simulink subsystem "ESD"  (R2021a)
settings: Solver=VariableStepAuto  StartTime=0.0  StopTime=10.0  RelTol=1e-3
values from neighbouring files (symbols this model uses):
  params = bestParams    [trainNet.m]
settings Model: Creator=trevor  LastModifiedBy=trevvvy
settings SolverCC: AlgebraicLoopSolver=TrustRegion
settings DebuggingCC: SFMachineParentedDataDiag=warning

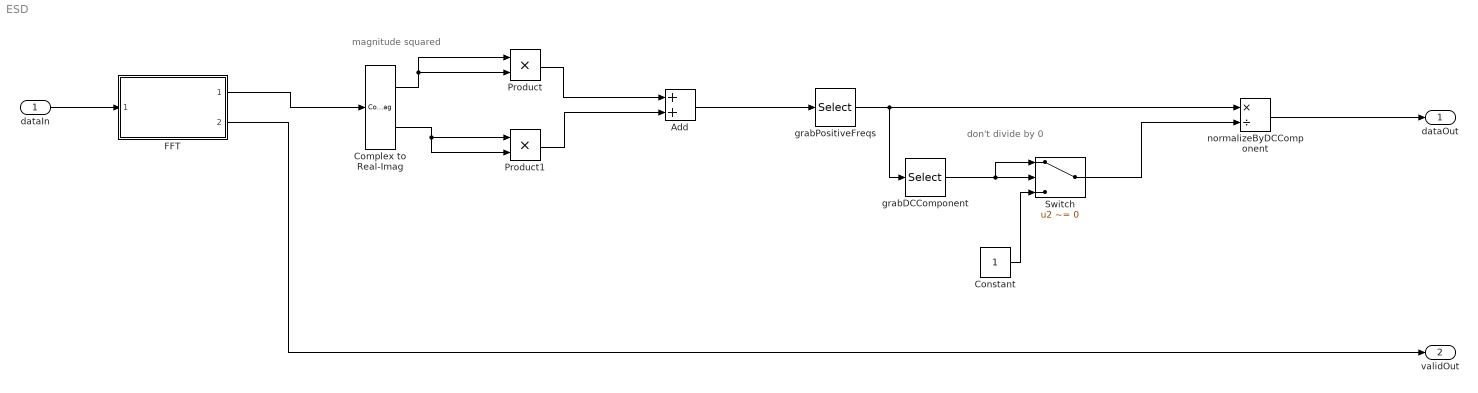
== system ESD ==
  note: don't divide by 0
  note: magnitude squared
  dataIn : Inport
  Add : Sum
  Complex to Real-Imag : ComplexToRealImag
  Constant : Constant  OutDataTypeStr=Inherit: Inherit via back propagation  SampleTime=-1
  FFT : Subsystem  ReferencedSubsystem=FFT
  Product : Product  OutDataTypeStr=Inherit: Same as first input
  Product1 : Product  OutDataTypeStr=Inherit: Same as first input
  Switch : Switch  Criteria=u2 ~= 0
  grabDCComponent : Selector  NumberOfDimensions=2  InputPortWidth=params.FFTSize  IndexOptions=Index vector (dialog),Index vector (dialog)  Indices=[1],1  OutputSizes=1,1
  grabPositiveFreqs : Selector  NumberOfDimensions=2  InputPortWidth=params.FFTSize  IndexOptions=Index vector (dialog),Index vector (dialog)  Indices=1,[1:params.FFTSize/2]  OutputSizes=1,1
  normalizeByDCComponent : Product  Inputs=*/  RndMeth=Zero  SaturateOnIntegerOverflow=on  OutDataTypeStr=Inherit: Same as first input
  dataOut : Outport
  validOut : Outport  Port=2
  wires:
  dataIn/1 -> FFT/1
  FFT/1 -> Complex to Real-Imag/1
  grabPositiveFreqs/1 -> normalizeByDCComponent/1, grabDCComponent/1
  grabDCComponent/1 -> Switch/2, Switch/1
  normalizeByDCComponent/1 -> dataOut/1
  Complex to Real-Imag/1 -> Product/1, Product/2
  Complex to Real-Imag/2 -> Product1/2, Product1/1
  Product1/1 -> Add/2
  Product/1 -> Add/1
  Add/1 -> grabPositiveFreqs/1
  Constant/1 -> Switch/3
  Switch/1 -> normalizeByDCComponent/2
  FFT/2 -> validOut/1
